simulink model "test_ROS_UDP"  (R2017b)
settings: Solver=FixedStepDiscrete  StartTime=0.0  StopTime=inf  FixedStep=0.1  RelTol=1e-3  EnableMultiTasking=on
libraries: instrumentlib x2, sldrtlib x1
settings Model: Creator=root  LastModifiedBy=Daniele
settings DataIOCC: LimitDataPoints=on  SaveFormat=Array  SignalLoggingSaveFormat=ModelDataLogs
settings OptimizationCC: ExpressionDepthLimit=2147483647  LifeSpan=inf
settings DebuggingCC: UnderspecifiedInitializationDetection=Classic  MergeDetectMultiDrivingBlocksExec=none  SolverPrmCheckMsg=warning  FcnCallInpInsideContextMsg=warning  StateNameClashWarn=warning  SFUnexpectedBacktrackingDiag=warning  SFNoUnconditionalDefaultTransitionDiag=warning  SFExecutionAtInitializationDiag=none
settings HardwareCC: ProdBitPerPointer=32  ProdBitPerSizeT=32  ProdBitPerPtrDiffT=32  ProdLargestAtomicFloat=None  ProdIntDivRoundTo=Undefined  ProdEndianess=Unspecified  ProdWordSize=32  ProdHWDeviceType=32-bit Generic
settings ModelReferenceCC: PropagateSignalLabelsOutOfModel=off
settings CodeAppCC: StateflowObjectComments=on
settings GRTTargetCC: TargetLangStandard=C89/C90 (ANSI)  GeneratePreprocessorConditionals=Disable all  CombineOutputUpdateFcns=off  GRTInterface=on
settings ConfigComp: CovMetricSettings=dw  CovHtmlReporting=on  CovSaveCumulativeToWorkspaceVar=on  CovSaveSingleToWorkspaceVar=on  CovExternalEMLEnable=off

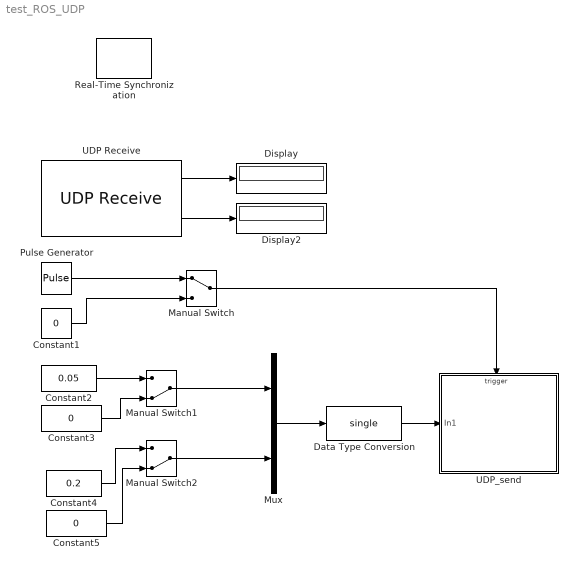
== system test_ROS_UDP ==
  Constant1 : Constant  Value=0
  Constant2 : Constant  Value=0.05
  Constant3 : Constant  Value=0
  Constant4 : Constant  Value=0.2
  Constant5 : Constant  Value=0
  Data Type Conversion : DataTypeConversion  OutDataTypeStr=single
  Display : Display
  Display2 : Display
  Manual Switch : ManualSwitch
  Manual Switch1 : ManualSwitch  CurrentSetting=0
  Manual Switch2 : ManualSwitch  CurrentSetting=0
  Mux : Mux  Inputs=2
  Pulse Generator : DiscretePulseGenerator  PulseType=Time based  Period=0.2  PulseWidth=50
  Real-Time Synchronization : sldrtlib/Real-Time Synchronization  SampleTime=0.1  MaxMissedTicks=10  ShowMissedTicks=off  YieldWhenWaiting=off
  UDP Receive : instrumentlib/UDP Receive  Host=192.168.1.7  Port=12002  LocalPort=12001  DataSize="[2  1]"  EnableBlockingMode=off  Timeout=10  SampleTime=0.1  DataType=single  ByteOrder=LittleEndian
      settings: SourceProductName=Instrument Control Toolbox
  UDP_send : Subsystem  TreatAsAtomicUnit=on
  wires:
  Pulse Generator/1 -> Manual Switch/1
  Constant1/1 -> Manual Switch/2
  Manual Switch/1 -> UDP_send/Trigger
  UDP Receive/1 -> Display/1
  UDP Receive/2 -> Display2/1
  Mux/1 -> Data Type Conversion/1
  Constant2/1 -> Manual Switch1/1
  Constant3/1 -> Manual Switch1/2
  Constant5/1 -> Manual Switch2/2
  Constant4/1 -> Manual Switch2/1
  Data Type Conversion/1 -> UDP_send/1(In1)
  Manual Switch1/1 -> Mux/1
  Manual Switch2/1 -> Mux/2

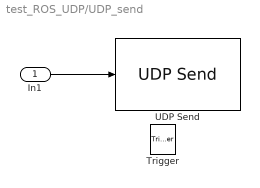
== system test_ROS_UDP/UDP_send ==
  In1 : Inport
  Trigger : TriggerPort  VariantControl=(inherit)
  UDP Send : instrumentlib/UDP Send  Host=192.168.1.7  Port=12002  LocalPort=12001  EnableBlockingMode=off  ByteOrder=LittleEndian
      settings: SourceProductName=Instrument Control Toolbox
  wires:
  In1/1 -> UDP Send/1
